simulink library "MPC_Sublibraries"  (R2020a)
settings: Solver=VariableStepAuto  StartTime=0.0  StopTime=10.0  RelTol=1e-3
(part 1 of 2)
settings Model: Creator=John Jr  LastModifiedBy=John Jr
settings SFSimCC: CustomCodeUndefinedFunction=UseInterfaceOnly

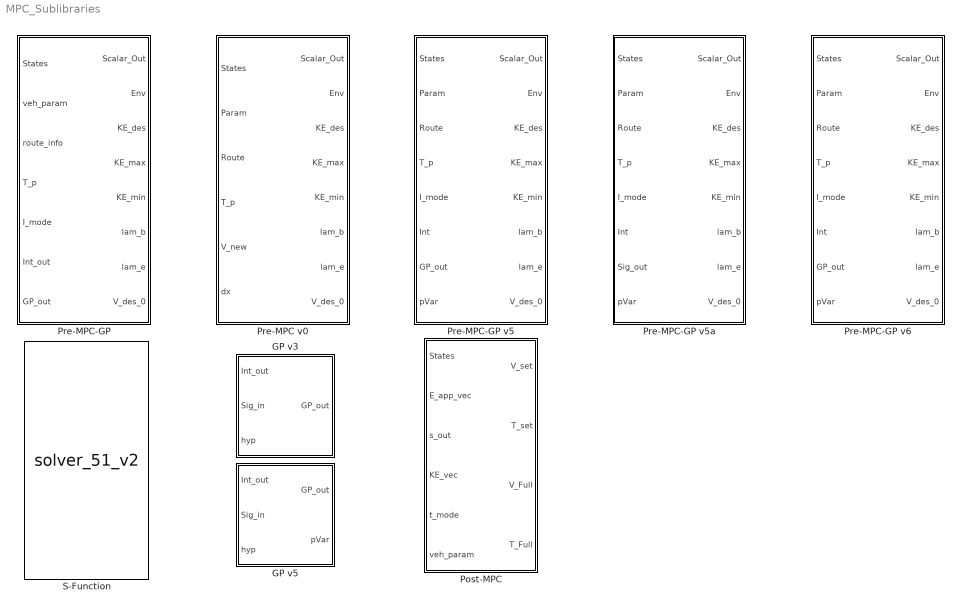
== system MPC_Sublibraries ==
  GP v3 : MATLAB Function  TreatAsAtomicUnit=on
  GP v5 : MATLAB Function  TreatAsAtomicUnit=on
  Post-MPC : MATLAB Function  TreatAsAtomicUnit=on
  Pre-MPC v0 : MATLAB Function  TreatAsAtomicUnit=on
  Pre-MPC-GP : MATLAB Function  TreatAsAtomicUnit=on
  Pre-MPC-GP v5 : MATLAB Function  TreatAsAtomicUnit=on
  Pre-MPC-GP v5a : MATLAB Function  TreatAsAtomicUnit=on
  Pre-MPC-GP v6 : MATLAB Function  TreatAsAtomicUnit=on
  S-Function : S-Function  FunctionName=solver_51_v2  SFunctionModules=solver_51_v2_wrapper  SFunctionDeploymentMode=off  EnableBusSupport=off
      mask Display:
      | patch([0 1 1 0], [0 0 1 1],[.8 1 1])
      | 
      | port_label('input',1,'\fontname{Cambria Math}Param','texmode','on')
      | port_label('input',2,'\fontname{Cambria Math}Env','texmode','on')
      | port_label('input',3,'\fontname{Cambria Math}KE_{des}','texmode','on')
      | port_label('input',4,'\fontname{Cambria Math}KE_{max}','texmode','on')
      | port_label('input',5,'\fontname{Cambria Math}KE_{min}','texmode','on')
      | port_label('input',6,'\fontname{Cambria Math}\lambda_b','texmode','on')
      | port_label('input',7,'\fontname{Cambria Math}\lambda_e','texmode','on')
      | 
      | port_label('output',1,'\fontname{Cambria Math}E_{app}','texmode','on')
      | port_label('output',2,'\fontname{Cambria Math}KE','texmode','on')
      | 
      | disp('\fontname{Cambria Math}\fontsize{14}Solver 51\newline      v2','texmode','on')

== matlab function MPC_Sublibraries/Pre-MPC-GP v5 ==
  data: States input size=4; Scalar_Out output; Env output size=51; Param input; Route input; T_p input; I_mode input; Int input; KE_des output size=51; KE_max output size=51; KE_min output size=51; lam_b output size=51; lam_e output size=51; V_des_0 output; GP_out input; pVar input
function [Scalar_Out,Env,KE_des,KE_max,KE_min,lam_b,lam_e,V_des_0] = ...
    fcn(States,Param,Route,T_p,I_mode,Int,GP_out,pVar)
%%  Extract Inputs
t_0 = States(3);                                        %   s - Sim time
x_0 = States(1);                                        %   m - Current position
v_0 = States(2);                                        %   m/s - Current velocity 
GR = States(4);                                         %   Current Gear
g = Param(1);                                           %   m/s^2 - Accel due to gravity
rho = Param(2);                                         %   kg/m^3 - Air density
m = Param(3);                                           %   kg - Base vehicle mass
Cd = Param(4);                                          %   Drag Coefficient
A_ref = Param(5);                                       %   m^2 - Reference area
Cr = Param(6);                                          %   Rolling resistance coefficient
r_wh = Param(7);                                        %   m - Wheel radius
X_vec = Route(:,1);                                     %   rad - Road grade angle vector
theta_vec = Route(:,2);                                 %   rad - Road grade angle vector
V_lim = Route(:,3);                                     %   m/s - Current speed limit
Int_cur = Int(:,1);                                     %   Current intersections within prediction horizon 
NI = length(Int_cur(~isnan(Int_cur(:,1)),1));           %   # of upcoming intersections 
Int_dx = Int(1:NI,2);                                   %   m - Distance to upcoming intersections 
Int_gap = Int(1:NI,3);                                  %   m - Intersection spacing 
L_0 = Int(1:NI,5);                                      %   Light status
B_0 = Int(1:NI,6);                                      %   Intersection minimum countdown time
tGR_vec = getGRvec_v5(Int,GP_out,pVar);                 %   Adjusted start time vectors
MI = length(tGR_vec(1:NI,:,1));                         %   # of future cycles considered 
[tGreen,~,tRed] = get_tCross1(tGR_vec,Int);             %   Time at which max green probability occurs
%%  Controller Setup
dx = 10;                                                %   m - Position step
NP = 51;                                                %   # of pred steps
x_pred = x_0+dx*NP-dx;                                  %   m - Prediction horizon length
XP = (linspace(x_0,x_pred,NP))';                        %   m - Position vector
a = 1;
%%  Horizon Vectors
V_des = zeros(NP,1);                                                %   m/s - Initialize des velocty vector
v_lim = interp1(X_vec,V_lim,XP,'previous',V_lim(end));              %   m/s - Maximum velocity vector 
v_min = 0*v_lim;                                                    %   m/s - Minimum velocity vector 
theta = interp1(X_vec,theta_vec,XP,'linear',theta_vec(end));        %   rad - Road grade vector 
KE_max = .5*m*v_lim.^2;                                             %   J - Maximum kinetic energy vector 
KE_min = .5*m*v_min.^2;                                             %   J - Minimum kinetic energy vector 
F_grav = m*g*sin(theta);                                            %   N - Gravitational force vector 
F_road = m*g*Cr*cos(theta);                                         %   N - Rolling resistance force vector 
Env = (F_road+F_grav)*dx;                                           %   J - Environmental resistance energy vector 
%%  Construct the desired velocity profile 
if I_mode == 1
    Int_x = x_0+Int_dx;                                             %   m - Intersection locations
    v_red = zeros(NI,1);                                            %   m/s - Initialize temp desired velocity vector
    v_des = zeros(NI,1);                                            %   m/s - Initialize temp desired velocity vector
    tC = zeros(NI,1);                                               %   s - Time at which v_des reaches the intersection 
    if NI == 1
        Int_v = interp1(X_vec,V_lim,...                             %   m/s - Intersection max velocity
            x_0,'linear',V_lim(end));
    else
        Int_v = interp1(X_vec,V_lim,...                             %   m/s - Intersection max velocity
            [x_0;Int_x(1:end-1)],'linear',V_lim(end));
    end
    for i = 1:NI
        if L_0(i) == 0 && tRed(i,1) <= t_0
            tRed(i,1) = t_0+B_0(i);
        end
        if i == 1   %%%%%%%%%%%%%%%%%%%%%%%%%%%%%%%%%%%%%%%%%%%%%%%%%   1st segment   %%%%%%%%%%%%%%%%%%%%%%%%%%%%%%%%%%%%%%%%%%%%%%%%
            t_star = a*tGreen(i,:)+(1-a)*tRed(i,:);                 %   Target crossing times 
            t_starR = tRed(i,:);                                    %   Red crossing time 
            v_star = Int_gap(i)./(t_star-t_0);                      %   Potential desired velocities 
            v_starR = Int_gap(i)./(t_starR-t_0);                    %   Potential backup desired velocities 
            Int_t = Int_gap(i)/Int_v(i)+t_0;                        %   Time at which speed limit reaches intersection 
            if (L_0(i) == 0 || L_0(i) == 1) && Int_t < tRed(1)...   %   Light is green and speed limit is still feasible even
                    && (v_star(1) > Int_v(i) || v_star(1) <= 0)     %   though the potential desired velocity isn't 
                v_des(i) = Int_v(i);
            else
                v_des(i) = max(v_star(v_star <= Int_v(i)));         %   First feasible velocity 
                v_red(i) = max(v_starR(v_starR <= Int_v(i)));       %   First feasible red velocity
                if v_red(i) > v_des(i)                              %   The earlier green window is still feasible to pass through 
                    v_des(i) = Int_v(i);                            %   Reassign the desired velocity 
                end
            end
            tC(i) = Int_gap(i)/v_des(i)+t_0;                        %   s - Time at which v_des reaches the intersection 
        else   %%%%%%%%%%%%%%%%%%%%%%%%%%%%%%%%%%%%%%%%%%%%%%%%%%%%%%   Remaining segments   %%%%%%%%%%%%%%%%%%%%%%%%%%%%%%%%%%%%%%%%%
            t_star = a*tGreen(i,:)+(1-a)*tRed(i,:);                 %   Target crossing times 
            t_starR = tRed(i,:);                                    %   Red crossing time
            v_star = Int_gap(i)./(t_star-tC(i-1));                  %   Potential desired velocities 
            v_starR = Int_gap(i)./(t_starR-tC(i-1));                %   Potential backup velocities 
            v_des(i) = max(v_star(v_star <= Int_v(i)));             %   First feasible velocity 
            v_red(i) = max(v_starR(v_starR <= Int_v(i)));           %   First feasible redvelocity
            if v_red(i) > v_des(i)                                  %   The earlier green window is still feasible to pass through
                v_des(i) = Int_v(i);                                %   Reassign the desired velocity
            end
            tC(i) = Int_gap(i)/v_des(i)+tC(i-1);                    %   s - Time at which v_des reaches the intersection 
        end
    end
    for i = 1:NP
        V_des(i) = interp1([x_0;Int_x],...                          %   m/s - Desired velocity through intersections 
            [v_des;v_des(end)],XP(i),'previous','extrap');
    end
else
    Int_x = NaN;
    for i = 1:NP
        V_des(i) = interp1(X_vec,V_lim,XP(i),...                    %   m/s - Desired velocity through intersections
            'linear',V_lim(end));
    end
end
%%  Prepare MPC parameters
V_des_0 = V_des(1);                                     %   m/s - 1st desired velocity 
A = 1-1/m*rho*Cd*A_ref*dx;                              %   Dynamics matrix
KE_0 = 1/2*m*v_0^2;                                     %   J - Initial kinetic energy 
F_wh_max = min(2200.*2.47*GR/r_wh,80000);               %   N - Maximum control force
E_mech_max = F_wh_max*dx;                               %   J - Initial max ME
E_mech_min = 0;                                         %   J - Mechanical energy lower limit 
E_brk_max = 35000*dx;                                   %   J - Brake energy upper limit 
E_brk_min = 0;                                          %   J - Brake energy lower limit 
U_p = T_p/r_wh*dx;                                      %   Previous control value
dU = 1e5;                                               %   J - Max control step
KE_des = 1/2*m.*V_des.^2;                               %   J - Initialize desired KE vector
lam_e = zeros(NP,1); lam_b = zeros(NP,1);               %   Initialize objective function weights 
[lam_e(:,1),lam_b(:,1)] = getWeights(XP,Int_x,I_mode);  %   Objective function weights

Scalar_Out = [A,KE_0,E_mech_max,E_mech_min,...
    E_brk_max,E_brk_min,U_p,dU]';

== matlab function MPC_Sublibraries/Pre-MPC-GP v5a ==
  data: States input size=4; Scalar_Out output; Env output size=51; Param input; Route input; T_p input; I_mode input; Int input; KE_des output size=51; KE_max output size=51; KE_min output size=51; lam_b output size=51; lam_e output size=51; V_des_0 output; Sig_out input; pVar input
function [Scalar_Out,Env,KE_des,KE_max,KE_min,lam_b,lam_e,V_des_0] = ...
    fcn(States,Param,Route,T_p,I_mode,Int,Sig_out,pVar)
%%  Extract Inputs
t_0 = States(3);                                        %   s - Sim time
x_0 = States(1);                                        %   m - Current position
v_0 = States(2);                                        %   m/s - Current velocity 
GR = States(4);                                         %   Current Gear
g = Param(1);                                           %   m/s^2 - Accel due to gravity
rho = Param(2);                                         %   kg/m^3 - Air density
m = Param(3);                                           %   kg - Base vehicle mass
Cd = Param(4);                                          %   Drag Coefficient
A_ref = Param(5);                                       %   m^2 - Reference area
Cr = Param(6);                                          %   Rolling resistance coefficient
r_wh = Param(7);                                        %   m - Wheel radius
X_vec = Route(:,1);                                     %   rad - Road grade angle vector
theta_vec = Route(:,2);                                 %   rad - Road grade angle vector
V_lim = Route(:,3);                                     %   m/s - Current speed limit
Int_cur = Int(:,1);                                     %   Current intersections within prediction horizon 
NI = length(Int_cur(~isnan(Int_cur(:,1)),1));           %   # of upcoming intersections 
Int_dx = Int(1:NI,2);                                   %   m - Distance to upcoming intersections 
Int_gap = Int(1:NI,3);                                  %   m - Intersection spacing 
L_0 = Int(1:NI,5);                                      %   Light status
B_0 = Int(1:NI,6);                                      %   Intersection minimum countdown time
tGR_vec = getGRvec_v5a(Int,Sig_out,pVar);               %   Adjusted start time vectors
MI = length(tGR_vec(1:NI,:,1));                         %   # of future cycles considered 
[tGreen,~,tRed] = get_tCross_v5a(tGR_vec,Int);          %   Time at which max green probability occurs
%%  Controller Setup
dx = 10;                                                %   m - Position step
NP = 51;                                                %   # of pred steps
x_pred = x_0+dx*NP-dx;                                  %   m - Prediction horizon length
XP = (linspace(x_0,x_pred,NP))';                        %   m - Position vector
a = 1;
%%  Horizon Vectors
V_des = zeros(NP,1);                                                %   m/s - Initialize des velocty vector
v_lim = interp1(X_vec,V_lim,XP,'previous',V_lim(end));              %   m/s - Maximum velocity vector 
v_min = 0*v_lim;                                                    %   m/s - Minimum velocity vector 
theta = interp1(X_vec,theta_vec,XP,'linear',theta_vec(end));        %   rad - Road grade vector 
KE_max = .5*m*v_lim.^2;                                             %   J - Maximum kinetic energy vector 
KE_min = .5*m*v_min.^2;                                             %   J - Minimum kinetic energy vector 
F_grav = m*g*sin(theta);                                            %   N - Gravitational force vector 
F_road = m*g*Cr*cos(theta);                                         %   N - Rolling resistance force vector 
Env = (F_road+F_grav)*dx;                                           %   J - Environmental resistance energy vector 
%%  Construct the desired velocity profile 
if I_mode == 1
    Int_x = x_0+Int_dx;                                             %   m - Intersection locations
    v_red = zeros(NI,1);                                            %   m/s - Initialize temp desired velocity vector
    v_des = zeros(NI,1);                                            %   m/s - Initialize temp desired velocity vector
    tC = zeros(NI,1);                                               %   s - Time at which v_des reaches the intersection 
    if NI == 1
        Int_v = interp1(X_vec,V_lim,...                             %   m/s - Intersection max velocity
            x_0,'linear',V_lim(end));
    else
        Int_v = interp1(X_vec,V_lim,...                             %   m/s - Intersection max velocity
            [x_0;Int_x(1:end-1)],'linear',V_lim(end));
    end
    for i = 1:NI
        if L_0(i) == 0 && tRed(i,1) <= t_0
            tRed(i,1) = t_0+B_0(i);
        end
        if i == 1   %%%%%%%%%%%%%%%%%%%%%%%%%%%%%%%%%%%%%%%%%%%%%%%%%   1st segment   %%%%%%%%%%%%%%%%%%%%%%%%%%%%%%%%%%%%%%%%%%%%%%%%
            t_star = a*tGreen(i,:)+(1-a)*tRed(i,:);                 %   Target crossing times 
            t_starR = tRed(i,:);                                    %   Red crossing time 
            v_star = Int_gap(i)./(t_star-t_0);                      %   Potential desired velocities 
            v_starR = Int_gap(i)./(t_starR-t_0);                    %   Potential backup desired velocities 
            Int_t = Int_gap(i)/Int_v(i)+t_0;                        %   Time at which speed limit reaches intersection 
            if (L_0(i) == 0 || L_0(i) == 1) && Int_t < tRed(1)...   %   Light is green and speed limit is still feasible even
                    && (v_star(1) > Int_v(i) || v_star(1) <= 0)     %   though the potential desired velocity isn't 
                v_des(i) = Int_v(i);
            else
                v_des(i) = max(v_star(v_star <= Int_v(i)));         %   First feasible velocity 
                v_red(i) = max(v_starR(v_starR <= Int_v(i)));       %   First feasible red velocity
                if v_red(i) > v_des(i)                              %   The earlier green window is still feasible to pass through 
                    v_des(i) = Int_v(i);                            %   Reassign the desired velocity 
                end
            end
            tC(i) = Int_gap(i)/v_des(i)+t_0;                        %   s - Time at which v_des reaches the intersection 
        else   %%%%%%%%%%%%%%%%%%%%%%%%%%%%%%%%%%%%%%%%%%%%%%%%%%%%%%   Remaining segments   %%%%%%%%%%%%%%%%%%%%%%%%%%%%%%%%%%%%%%%%%
            t_star = a*tGreen(i,:)+(1-a)*tRed(i,:);                 %   Target crossing times 
            t_starR = tRed(i,:);                                    %   Red crossing time
            v_star = Int_gap(i)./(t_star-tC(i-1));                  %   Potential desired velocities 
            v_starR = Int_gap(i)./(t_starR-tC(i-1));                %   Potential backup velocities 
            v_des(i) = max(v_star(v_star <= Int_v(i)));             %   First feasible velocity 
            v_red(i) = max(v_starR(v_starR <= Int_v(i)));           %   First feasible redvelocity
            if v_red(i) > v_des(i)                                  %   The earlier green window is still feasible to pass through
                v_des(i) = Int_v(i);                                %   Reassign the desired velocity
            end
            tC(i) = Int_gap(i)/v_des(i)+tC(i-1);                    %   s - Time at which v_des reaches the intersection 
        end
    end
    for i = 1:NP
        V_des(i) = interp1([x_0;Int_x],...                          %   m/s - Desired velocity through intersections 
            [v_des;v_des(end)],XP(i),'previous','extrap');
    end
else
    Int_x = NaN;
    for i = 1:NP
        V_des(i) = interp1(X_vec,V_lim,XP(i),...                    %   m/s - Desired velocity through intersections
            'linear',V_lim(end));
    end
end
%%  Prepare MPC parameters
V_des_0 = V_des(1);                                     %   m/s - 1st desired velocity 
A = 1-1/m*rho*Cd*A_ref*dx;                              %   Dynamics matrix
KE_0 = 1/2*m*v_0^2;                                     %   J - Initial kinetic energy 
F_wh_max = min(2200.*2.47*GR/r_wh,80000);               %   N - Maximum control force
E_mech_max = F_wh_max*dx;                               %   J - Initial max ME
E_mech_min = 0;                                         %   J - Mechanical energy lower limit 
E_brk_max = 35000*dx;                                   %   J - Brake energy upper limit 
E_brk_min = 0;                                          %   J - Brake energy lower limit 
U_p = T_p/r_wh*dx;                                      %   Previous control value
dU = 1e5;                                               %   J - Max control step
KE_des = 1/2*m.*V_des.^2;                               %   J - Initialize desired KE vector
lam_e = zeros(NP,1); lam_b = zeros(NP,1);               %   Initialize objective function weights 
[lam_e(:,1),lam_b(:,1)] = getWeights(XP,Int_x,I_mode);  %   Objective function weights

Scalar_Out = [A,KE_0,E_mech_max,E_mech_min,...
    E_brk_max,E_brk_min,U_p,dU]';

== matlab function MPC_Sublibraries/Pre-MPC-GP v6 ==
  data: States input size=4; Scalar_Out output; Env output size=51; Param input; Route input; T_p input; I_mode input; Int input; KE_des output size=51; KE_max output size=51; KE_min output size=51; lam_b output size=51; lam_e output size=51; V_des_0 output; GP_out input; pVar input
function [Scalar_Out,Env,KE_des,KE_max,KE_min,lam_b,lam_e,V_des_0] = ...
    fcn(States,Param,Route,T_p,I_mode,Int,GP_out,pVar)
%%  Extract Inputs
t_0 = States(3);                                        %   s - Sim time
x_0 = States(1);                                        %   m - Current position
v_0 = States(2);                                        %   m/s - Current velocity 
GR = States(4);                                         %   Current Gear
g = Param(1);                                           %   m/s^2 - Accel due to gravity
rho = Param(2);                                         %   kg/m^3 - Air density
m = Param(3);                                           %   kg - Base vehicle mass
Cd = Param(4);                                          %   Drag Coefficient
A_ref = Param(5);                                       %   m^2 - Reference area
Cr = Param(6);                                          %   Rolling resistance coefficient
r_wh = Param(7);                                        %   m - Wheel radius
X_vec = Route(:,1);                                     %   rad - Road grade angle vector
theta_vec = Route(:,2);                                 %   rad - Road grade angle vector
V_lim = Route(:,3);                                     %   m/s - Current speed limit
Int_cur = Int(:,1);                                     %   Current intersections within prediction horizon 
NI = length(Int_cur(~isnan(Int_cur(:,1)),1));           %   # of upcoming intersections 
Int_dx = Int(1:NI,2);                                   %   m - Distance to upcoming intersections 
Int_gap = Int(1:NI,3);                                  %   m - Intersection spacing 
L_0 = Int(1:NI,5);                                      %   Light status
B_0 = Int(1:NI,6);                                      %   Intersection minimum countdown time
tGR_vec = getGRvec_v5(Int,GP_out,pVar);                 %   Adjusted start time vectors
MI = length(tGR_vec(1:NI,:,1));                         %   # of future cycles considered 
[tGreen,~,tRed] = get_tCross1(tGR_vec,Int);             %   Time at which max green probability occurs
%%  Controller Setup
dx = 10;                                                %   m - Position step
NP = 51;                                                %   # of pred steps
x_pred = x_0+dx*NP-dx;                                  %   m - Prediction horizon length
XP = (linspace(x_0,x_pred,NP))';                        %   m - Position vector
a = 1;
%%  Horizon Vectors
V_des = zeros(NP,1);                                                %   m/s - Initialize des velocty vector
v_lim = interp1(X_vec,V_lim,XP,'previous',V_lim(end));              %   m/s - Maximum velocity vector 
v_min = 0*v_lim;                                                    %   m/s - Minimum velocity vector 
theta = interp1(X_vec,theta_vec,XP,'linear',theta_vec(end));        %   rad - Road grade vector 
KE_max = .5*m*v_lim.^2;                                             %   J - Maximum kinetic energy vector 
KE_min = .5*m*v_min.^2;                                             %   J - Minimum kinetic energy vector 
F_grav = m*g*sin(theta);                                            %   N - Gravitational force vector 
F_road = m*g*Cr*cos(theta);                                         %   N - Rolling resistance force vector 
Env = (F_road+F_grav)*dx;                                           %   J - Environmental resistance energy vector 
%%  Construct the desired velocity profile 
if I_mode == 1
    Int_x = x_0+Int_dx;                                             %   m - Intersection locations
    v_red = zeros(NI,1);                                            %   m/s - Initialize temp desired velocity vector
    v_des = zeros(NI,1);                                            %   m/s - Initialize temp desired velocity vector
    tC = zeros(NI,1);                                               %   s - Time at which v_des reaches the intersection 
    if NI == 1
        Int_v = interp1(X_vec,V_lim,...                             %   m/s - Intersection max velocity
            x_0,'linear',V_lim(end));
    else
        Int_v = interp1(X_vec,V_lim,...                             %   m/s - Intersection max velocity
            [x_0;Int_x(1:end-1)],'linear',V_lim(end));
    end
    for i = 1:NI
        if L_0(i) == 0 && tRed(i,1) <= t_0
            tRed(i,1) = t_0+B_0(i);
        end
        if i == 1   %%%%%%%%%%%%%%%%%%%%%%%%%%%%%%%%%%%%%%%%%%%%%%%%%   1st segment   %%%%%%%%%%%%%%%%%%%%%%%%%%%%%%%%%%%%%%%%%%%%%%%%
            t_star = a*tGreen(i,:)+(1-a)*tRed(i,:);                 %   Target crossing times 
            t_starR = tRed(i,:);                                    %   Red crossing time 
            v_star = Int_gap(i)./(t_star-t_0);                      %   Potential desired velocities 
            v_starR = Int_gap(i)./(t_starR-t_0);                    %   Potential backup desired velocities 
            Int_t = Int_gap(i)/Int_v(i)+t_0;                        %   Time at which speed limit reaches intersection 
            if (L_0(i) == 0 || L_0(i) == 1) && Int_t < tRed(1)...   %   Light is green and speed limit is still feasible even
                    && (v_star(1) > Int_v(i) || v_star(1) <= 0)     %   though the potential desired velocity isn't 
                v_des(i) = Int_v(i);
            else
                v_des(i) = max(v_star(v_star <= Int_v(i)));         %   First feasible velocity 
                v_red(i) = max(v_starR(v_starR <= Int_v(i)));       %   First feasible red velocity
                if v_red(i) > v_des(i)                              %   The earlier green window is still feasible to pass through 
                    v_des(i) = Int_v(i);                            %   Reassign the desired velocity 
                end
            end
            tC(i) = Int_gap(i)/v_des(i)+t_0;                        %   s - Time at which v_des reaches the intersection 
        else   %%%%%%%%%%%%%%%%%%%%%%%%%%%%%%%%%%%%%%%%%%%%%%%%%%%%%%   Remaining segments   %%%%%%%%%%%%%%%%%%%%%%%%%%%%%%%%%%%%%%%%%
            t_star = a*tGreen(i,:)+(1-a)*tRed(i,:);                 %   Target crossing times 
            t_starR = tRed(i,:);                                    %   Red crossing time
            v_star = Int_gap(i)./(t_star-tC(i-1));                  %   Potential desired velocities 
            v_starR = Int_gap(i)./(t_starR-tC(i-1));                %   Potential backup velocities 
            v_des(i) = max(v_star(v_star <= Int_v(i)));             %   First feasible velocity 
            v_red(i) = max(v_starR(v_starR <= Int_v(i)));           %   First feasible redvelocity
            if v_red(i) > v_des(i)                                  %   The earlier green window is still feasible to pass through
                v_des(i) = Int_v(i);                                %   Reassign the desired velocity
            end
            tC(i) = Int_gap(i)/v_des(i)+tC(i-1);                    %   s - Time at which v_des reaches the intersection 
        end
    end
    for i = 1:NP
        V_des(i) = interp1([x_0;Int_x],...                          %   m/s - Desired velocity through intersections 
            [v_des;v_des(end)],XP(i),'previous','extrap');
    end
else
    Int_x = NaN;
    for i = 1:NP
        V_des(i) = interp1(X_vec,V_lim,XP(i),...                    %   m/s - Desired velocity through intersections
            'linear',V_lim(end));
    end
end
%%  Prepare MPC parameters
V_des_0 = V_des(1);                                     %   m/s - 1st desired velocity 
A = 1-1/m*rho*Cd*A_ref*dx;                              %   Dynamics matrix
KE_0 = 1/2*m*v_0^2;                                     %   J - Initial kinetic energy 
F_wh_max = min(2200.*2.47*GR/r_wh,80000);               %   N - Maximum control force
E_mech_max = F_wh_max*dx;                               %   J - Initial max ME
E_mech_min = 0;                                         %   J - Mechanical energy lower limit 
E_brk_max = 35000*dx;                                   %   J - Brake energy upper limit 
E_brk_min = 0;                                          %   J - Brake energy lower limit 
U_p = T_p/r_wh*dx;                                      %   Previous control value
dU = 1e5;                                               %   J - Max control step
KE_des = 1/2*m.*V_des.^2;                               %   J - Initialize desired KE vector
lam_e = zeros(NP,1); lam_b = zeros(NP,1);               %   Initialize objective function weights 
[lam_e(:,1),lam_b(:,1)] = getWeights_v6(XP,Int_x,I_mode);  %   Objective function weights

Scalar_Out = [A,KE_0,E_mech_max,E_mech_min,...
    E_brk_max,E_brk_min,U_p,dU]';

== matlab function MPC_Sublibraries/Post-MPC ==
  data: V_set output size=1; T_set output size=1; States input size=4; E_app_vec input; s_out input; KE_vec input; t_mode input; veh_param input; V_Full output; T_Full output
function [V_set,T_set,V_Full,T_Full] = fcn(States,...
    E_app_vec,s_out,KE_vec,t_mode,veh_param)

m = veh_param(3);                                   %   kg - Base vehicle mass
r_wh = veh_param(7);                                %   m - Wheel radius
v_0 = States(2);
t_0 = States(3);

nc_steps = length(KE_vec);
dx = 10;
KE = zeros(1,nc_steps);
U_app_ref = E_app_vec/dx; 
KE(1) = s_out(2);
for i = 2:nc_steps
    KE(i) = KE_vec(i-1);
    if KE(i) < 0
        KE(i) = 0;
    end
end
V_ref = sqrt(2/m*KE);
t_ref = t_0*ones(1,nc_steps); 
for i = 2:nc_steps
    if mean([V_ref(i) V_ref(i-1)]) < .1
        t_ref(i) = t_ref(i-1)+dx/.1;
    else
        t_ref(i) = t_ref(i-1)+dx/mean([V_ref(i) V_ref(i-1)]);
    end
end

if t_mode == 1
    dt = 1;                                         %   Time step
    t_vec = 0:1:24;                                 %   Horizon time vector
else
    dt = 5;                                         %   Time step
    t_vec = 0:5:120;                                %   Horizon time vector
end
np_steps = length(t_vec);    
U_app = zeros(1,np_steps);                          %   N - Initialize control force vector       
t = t_0*ones(1,np_steps);                           %   N - Initialize time vector
V = zeros(1,np_steps);                              %   m/s - Initialize velocity vector

U_app(1) = U_app_ref(1);
V(1) = v_0;                                         %   m/s - Initial velocity

for i = 2:np_steps
    t(i) = t(i-1)+dt;
    U_app(i) = interp1(t_ref,U_app_ref,t(i),...
        'previous','extrap');
    V(i) = interp1(t_ref,V_ref,t(i),...
        'linear','extrap');
end
V_set = V(2);
T_set = U_app(1)*r_wh;
V_Full = V';
T_Full = U_app(1:end-1)'*r_wh;

== matlab function MPC_Sublibraries/GP v5 ==
  data: Int_out input; Sig_in input; GP_out output; hyp input; pVar output
function [GP_out,pVar] = GP_v4(Int_out,Sig_in,hyp)

L_0 = Int_out(:,5);                             %   What is known
N = length(Sig_in(~isnan(Sig_in(:,1,1))));      %   # of intersections 
M = length(Sig_in(:,1,1));                      %   # of temp placeholders
m = 7;                                          %   # of future predictions
GP_out = NaN*ones(M,m,4);                       %   Predicted mean and variances:   (:,:,1) -> G_p; (:,:,3) -> G_v
                                                %                                   (:,:,2) -> R_p; (:,:,4) -> R_v
pVar = zeros(m,m,M,2);                          %   Prediction variance matrices 
for i = 1:N
    xG = Sig_in(i,:,3)';                        %   Past cycle numbers with known green phase lengths
    xR = Sig_in(i,:,4)';                        %   Past cycle numbers with known red phase lengths
    G_vec = Sig_in(i,:,1);                      %   Past green phase lengths
    R_vec = Sig_in(i,:,2);                      %   Past red phase lengths
    if L_0(i) == 0
        mG = m;     mR = m;                     %   # of future predictions required for each phase color
    elseif L_0(i) == 3
        mG = m-1;   mR = m-1;                   %   # of future predictions required for each phase color
        GP_out(i,1:2,1) = G_vec(end-1:end);     %   Current green phase length is known
        GP_out(i,1:2,3) = 0;                    %   Current green phase length variance = 0
        GP_out(i,1,2) = R_vec(end);             %   Current red phase length is known
        GP_out(i,1,4) = 0;                      %   Current red phase length variance = 0
    else
        mG = m-1;     mR = m;                   %   # of future predictions required for each phase color
        GP_out(i,1,1) = G_vec(end);             %   Current green phase length is known
        GP_out(i,1,3) = 0;                      %   Current green phase length variance = 0
    end
    rG = m-mG+1:m;  rR = m-mR+1:m;              %   Output reference ranges
    xGs = (xG(end)+1:xG(end)+mG)';              %   Future cycle numbers for green phase lengths
    xRs = (xR(end)+1:xR(end)+mR)';              %   Future cycle numbers for red phase lengths
    [G_p,G_v,pGV] =...                          %   Run GP for green phase lengths
        myGP_v5(xG,xGs,G_vec,hyp(i,:,1));
    [R_p,R_v,pRV] =...                          %   Run GP for red phase lengths
        myGP_v5(xR,xRs,R_vec,hyp(i,:,2));
    GP_out(i,rG,1) = G_p';                      %   Predicted green phase lengths
    GP_out(i,rG,3) = G_v';                      %   Predicted variance for green phase lengths
    GP_out(i,rR,2) = R_p';                      %   Predicted green phase lengths
    GP_out(i,rR,4) = R_v';                      %   Predicted variance for green phase lengths
    pVar(rG,rG,i,1) = pGV;                      %   Prediction variance matrices for green phase lengths 
    pVar(rR,rR,i,2) = pRV;                      %   Prediction variance matrices for red phase lengths
end
end

== matlab function MPC_Sublibraries/Pre-MPC-GP ==
  data: States input size=4; Scalar_Out output; Env output size=51; veh_param input; route_info input; T_p input; I_mode input; Int_out input; KE_des output size=51; KE_max output size=51; KE_min output size=51; lam_b output size=51; lam_e output size=51; V_des_0 output; GP_out input
function [Scalar_Out,Env,KE_des,KE_max,KE_min,lam_b,lam_e,V_des_0] = ...
    fcn(States,veh_param,route_info,T_p,I_mode,Int_out,GP_out)
%%  
t_0 = States(3);                                        %   s - Sim time
x_0 = States(1);                                        %   m - Current position
v_0 = States(2);                                        %   m/s - Current velocity 
GR = States(4);                                         %   Current Gear
g = veh_param(1);                                       %   m/s^2 - Accel due to gravity
rho = veh_param(2);                                     %   kg/m^3 - Air density
m = veh_param(3);                                       %   kg - Base vehicle mass
Cd = veh_param(4);                                      %   Drag Coefficient
A_ref = veh_param(5);                                   %   m^2 - Reference area
Cr = veh_param(6);                                      %   Rolling resistance coefficient
r_wh = veh_param(7);                                    %   m - Wheel radius
X_vec = route_info(:,1);                                %   rad - Road grade angle vector
theta_vec = route_info(:,2);                            %   rad - Road grade angle vector
V_lim = route_info(:,3);                                %   m/s - Current speed limit
% v_DP = route_info(:,4);                                 %   m/s - Offline optimized velocity                                       


%%  Controller Setup
dx = 10;                                                %   m - Position step
N = 51;                                                 %   # of pred steps
x_pred = x_0+dx*N-dx;                                   %   m - Prediction horizon length
xp_vec = (linspace(x_0,x_pred,N))';                     %   m - Position vector

%%  Horizon Vectors
V_des = zeros(N,1);                                                 %   m/s - Initialize des velocty vector
V_des_0 = 0;                                                        %   m/s - Initialize 1st desired velocity
v_lim = interp1(X_vec,V_lim,xp_vec,'linear',V_lim(end));            %   m/s - Maximum velocity vector 
v_min = 0*v_lim;                                                    %   m/s - Minimum velocity vector 
theta = interp1(X_vec,theta_vec,xp_vec,'linear',theta_vec(end));    %   rad - Road grade vector 
KE_max = .5*m*v_lim.^2;                                             %   J - Maximum kinetic energy vector 
KE_min = .5*m*v_min.^2;                                             %   J - Minimum kinetic energy vector 
F_grav = m*g*sin(theta);                                            %   N - Gravitational force vector 
F_road = m*g*Cr*cos(theta);                                         %   N - Rolling resistance force vector 
Env = (F_road+F_grav)*dx;                                           %   J - Environmental resistance energy vector 

%%  Intersection properties
if I_mode == 1
    [G_in,R_in,t_g,tg_v,t_r,tr_v] = getGRvec_v3(Int_out,GP_out);    %   Get start times for predicted green and red phases 
    NI = length(Int_out(isnan(Int_out(:,1))==0));                   %   # of upcoming intersections
    M = length(G_in(1,:));                                          %   # of green and red times
    CI_check = zeros(NI,M);                                         %   Check if probability of green is above 95%
    pGreen = zeros(NI,M);                                           %   Probability of green 
    tGreen = zeros(NI,M);                                           %   s - Time at which green probability is highest 
    tRed = zeros(NI,M);                                             %   s - Time at which red light turns red
    Int_dx = zeros(NI,1);                                           %   m - Initialize distance to intersections vector 
    Int_ds = zeros(NI,1);                                           %   m - Initialize distance between intersections vector 
    G = zeros(NI,M);                                                %   m - Initialize green time vector 
    R = zeros(NI,M);                                                %   m - Initialize red time vector 
    for i = 1:NI
        for j = 1:M
            if R_in(i,j) < G_in(i,j)                        %   Probability of green is less than 95%
                CI_check(i,j) = 1;                          %   Set jth index to 1 
            elseif R_in(i,j) == G_in(i,j)                           %   Probability of green is equal to 95%
                tGreen(i,j) = G_in(i,j);                            %   s - Target green time
                tRed(i,j) = R_in(i,j);                              %   s - Time light turns red
                pGreen(i,j) = .95;                                  %   Probability of green 
            else                                                    %   Probability of green is above 95%
                tGreen(i,j) = mean([G_in(i,j),R_in(i,j)]);          %   s - Target green time
                tRed(i,j) = R_in(i,j);                              %   s - Time light turns red
                pGreen(i,j) = 1;                                    %   Probability of green 
            end
        end
        index1 = find(CI_check(i,:) == 1);                          %   Green intervals that need to be investigated further
        if ~isempty(index1)
            [tG,pG] = getProb_v3(i,Int_out,GP_out,t_g,...           %   Obtain remaining green times and corresponding probability 
                tg_v,t_r,tr_v,index1);
            tGreen(i,index1) = tG;                                  %   s - Target green time
            tRed(i,index1) = tG;                                    %   s - Time light turns red
            pGreen(i,index1) = pG;                                  %   Probability of green 
        end
        Int_dx(i) = Int_out(i,2);                                   %   m - Distance to intersections
        Int_ds(i) = Int_out(i,3);                                   %   m - Distance between intersections
        G(i,:) = G_in(i,:);                                         %   s - Time light turns green
        R(i,:) = R_in(i,:);                                         %   s - Time light turns red
    end
    Int_x = x_0+Int_dx;                                             %   m - Intersection locations
    C_cur = zeros(NI,1);
    Red_Light = zeros(NI,1);                                        %   Initialize red light vector
    v_max_adj = zeros(NI,1);                                %   m/s - Initialize max vel adj vector
    v_min_adj = zeros(NI,1);                                %   m/s - Initialize min vel adj vector
    v_des = zeros(NI,1);                                    %   m/s - Initialize desired velocity vector
    G_dt = zeros(NI,M);                                     %   s - Time to green
    G_dt1 = zeros(NI,M);                                    %   s - Time to green
    v_max_G = zeros(NI,M);                                  %   m/s - Velocity to reach light at green 
    v_max_G1 = zeros(NI,M);                                 %   m/s - Velocity to reach light at green 
    R_dt = zeros(NI,M);                                     %   s - Time to red
    v_min_R = zeros(NI,M);                                  %   m/s - Velocity to reach light at red 
    if NI == 1
        Int_v_max = interp1(X_vec,V_lim,...                     %   m/s - Intersection max velocity
            x_0,'linear',V_lim(end));
    else
        Int_v_max = interp1(X_vec,V_lim,...                     %   m/s - Intersection max velocity
            [x_0;Int_x(1:end-1)],'linear',V_lim(end));
    end
    Int_v_min = Int_v_max*.25;                              %   m/s - Intersection min velocity
    Int_t = t_0*ones(NI+1,1);                               %   s - Temp time vector for des vel
    Int_t_max = t_0*ones(NI+1,1);                           %   s - Temp time vector for max vel
    Int_t_min = t_0*ones(NI+1,1);                           %   s - Temp time vector for min vel
    for i = 1:NI
        C_cur(i) = find(Int_t(i) > G(i,:),1,'last');        %   s - Current light period
        if Int_t(i) < R(i,C_cur(i))                         %   Check current light status
            Red_Light(i) = 0;                               %   Light is green
        else
            Red_Light(i) = 1;                               %   Light is red
        end
        Int_condition = 0;                                  %   Initialize condition
        j = 0;                                              %   Initialize counter
        while Int_condition == 0                            %   Loop until feasible green intervals are found 
            j = j+1;                                        %   Increment counter
            if j == M+1                                     %   No feasible green intervals found
                Int_v_min(i) = max(Int_v_min(i)-1,0);       %   Decrement min velocity 
                j = 1;                                      %   Reset counter
            end
            G_dt(i,j) = G(i,j)-Int_t(i);                    %   s - Time till light turns green
            v_max_G(i,j) = Int_ds(i)/G_dt(i,j);             %   m/s - Velocity to reach li ght turning green
            G_dt1(i,j) = tGreen(i,j)-Int_t(i);              %   s - Time till light turns green
            v_max_G1(i,j) = Int_ds(i)/G_dt1(i,j);           %   m/s - Velocity to reach li ght turning green
            R_dt(i,j) = R(i,j)-Int_t(i);                    %   s - Time till light turns red
            v_min_R(i,j) = Int_ds(i)/R_dt(i,j);             %   m/s - Velocity to reach light turning red
            if Red_Light(i) == 0 && j == 1 ...              %   Light is green and on first cycle 
                    && v_min_R(i,j) < Int_v_max(i)...       %   Velocity to reach intersection at red is feasible 
                    && v_min_R(i,j) > 0                     %   Velocity to reach intersection at red is positive 
                Int_condition = 1;
                v_max_adj(i) = Int_v_max(i);                %   m/s - Adjusted maximum velocity
                v_min_adj(i) = max(v_max_G1(i,j)...         %   m/s - Adjusted minimum velocity
                    ,Int_v_min(i));
                v_des(i) = Int_v_max(i);                    %   m/s - Desired velocity 
            elseif v_max_G1(i,j) > Int_v_min(i)...          %   Velocity to reach intersection at green is above min velocity 
                    && v_max_G1(i,j) < Int_v_max(i)         %   Velocity to reach intersection at green is below max velocity 
                Int_condition = 2;
                v_max_adj(i) = min(Int_v_max(i)...          %   m/s - Adjusted minimum velocity
                    ,v_max_G1(i,j));
                v_min_adj(i) = v_max_G1(i,j);               %   m/s - Adjusted minimum velocity
                v_des(i) = v_max_G1(i,j);                   %   m/s - Desired velocity 
            elseif v_max_G1(i,j) < Int_v_max(i)...          %   Velocity to reach intersection at green is below max velocity 
                    && v_max_G1(i,j) > Int_v_min(i)
                Int_condition = 4;
                v_max_adj(i) = v_max_G1(i,j);               %   m/s - Adjusted minimum velocity
                v_min_adj(i) = max(Int_v_min(i),...         %   m/s - Adjusted minimum velocity
                    v_max_G1(i,j));        
                v_des(i) = v_max_G1(i,j);                   %   m/s - Desired velocity 
            end
        end
        Int_t(i+1) = Int_ds(i)/v_des(i)+Int_t(i);           %   s - Desired velocity time vector
        Int_t_max(i+1) = Int_ds(i)/v_max_adj(i)...          %   s - Max velocity time vector
            +Int_t_max(i);
        Int_t_min(i+1) = Int_ds(i)/v_min_adj(i)...          %   s - Min velocity time vector
            +Int_t_min(i); 
    end
    for i = 1:N
        V_des(i) = interp1([x_0;Int_x],...                  %   m/s - Desired velocity through intersections 
            [v_des;v_des(end)],xp_vec(i),...
            'previous','extrap');
        V_des_0 = V_des(1);                                 
    end
else
    Int_x = NaN;
    for i = 1:N
%         V_des(i) = interp1(X_vec,v_DP,xp_vec(i),...
%             'linear',v_DP(end));
        V_des(i) = interp1(X_vec,V_lim,xp_vec(i),...
            'linear',V_lim(end))*.9;
        V_des_0 = V_des(1);
    end
end
%%  Prepare NPC parameters
A = 1-1/m*rho*Cd*A_ref*dx;                              %   Dynamics matrix
KE_0 = 1/2*m*v_0^2;                                     %   J - Initial kinetic energy 
F_wh_max = min(2200.*2.47*GR/r_wh,80000);               %   N - Maximum control force
E_mech_max = F_wh_max*dx;                               %   J - Initial max ME
E_mech_min = 0;                                         %   J - Mechanical energy lower limit 
E_brk_max = 35000*dx;                                   %   J - Brake energy upper limit 
E_brk_min = 0;                                          %   J - Brake energy lower limit 
U_p = T_p/r_wh*dx;                                      %   Previous control value
dU = 1e5;                                               %   J - Max control step
KE_des = 1/2*m.*V_des.^2;                               %   J - Initialize desired KE vector
lam_e = zeros(N,1); lam_b = zeros(N,1);
[lam_e(:,1),lam_b(:,1)] = getWeights(xp_vec,Int_x,I_mode);        %   Objective weights

Scalar_Out = [A,KE_0,E_mech_max,E_mech_min,...
    E_brk_max,E_brk_min,U_p,dU]';

== matlab function MPC_Sublibraries/GP v3 ==
  data: Int_out input; Sig_in input; GP_out output; hyp input
function GP_out = GP_v3(Int_out,Sig_in,hyp)

L_0 = Int_out(:,5);                             %   s - Cycle start times
N = length(Sig_in(~isnan(Sig_in(:,1,1))));      %   # of intersections 
M = length(Sig_in(:,1,1));                      %   # of temp placeholders
n = length(Sig_in(1,:,1));                      %   # of past data points
m = 6;                                          %   # of future predictions
GP_out = NaN*ones(M,m,4);                       %   Predicted mean and variances:   (:,:,1) -> G_pred; (:,:,3) -> G_var
                                                %                                   (:,:,2) -> R_pred; (:,:,4) -> R_var
x = (1:n)';                                     %   Training data points vector
xStar1 = (n+1:n+m)';                            %   Candidate data points vector for unknown current phase
xStar2 = (n+1:n+m-1)';                          %   Candidate data points vector for known current phase
for i = 1:N
    G_vec = Sig_in(i,:,1);                              %   Past green phase lengths 
    R_vec = Sig_in(i,:,2);                              %   Past red phase lengths
    %   Green prediction 
    if L_0(i) == 0
        [GP_out(i,:,1),GP_out(i,:,3)] = myGP(x,...      %   Run GP for all green phases
            xStar1,G_vec,hyp(i,:,2));
    else
        GP_out(i,1,1) = G_vec(end);                     %   Current green phase is known
        GP_out(i,1,3) = 0;                              %   Therefore variance is zero
        [GP_out(i,2:m,1),GP_out(i,2:m,3)] = myGP(x,...  %   Run GP for remaining green phases
            xStar2,G_vec,hyp(i,:,2));
    end
    %   Red prediction
    if L_0(i) == 3
        GP_out(i,1,2) = R_vec(end);                     %   Current red phase is known
        GP_out(i,1,4) = 0;                              %   Therefore variance is zero
        [GP_out(i,2:m,2),GP_out(i,2:m,4)] = myGP(x,...  %   Run GP for remaining red phases
            xStar2,R_vec,hyp(i,:,3));
    else
        [GP_out(i,:,2),GP_out(i,:,4)] = myGP(x,...      %   Run GP for all red phases
            xStar1,R_vec,hyp(i,:,3));
    end
end
end
